simulink model "Regulation_Case"  (R2021a)
settings: Solver=VariableStepAuto  StartTime=0.0  StopTime=300  RelTol=1e-3
values from neighbouring files (symbols this model uses):
  kd = 500    [Parameters.m]
  kp = 50    [Parameters.m]
  omega0 = pi/180*[0.53 0.53 0.053]'    [Parameters.m]
  q0 = [0.6853 0.6953 0.1531 0.1531]'    [Parameters.m]
  qc = [0 0 0 1]'    [Parameters.m]
settings Model: Creator=VTX  LastModifiedBy=VTX

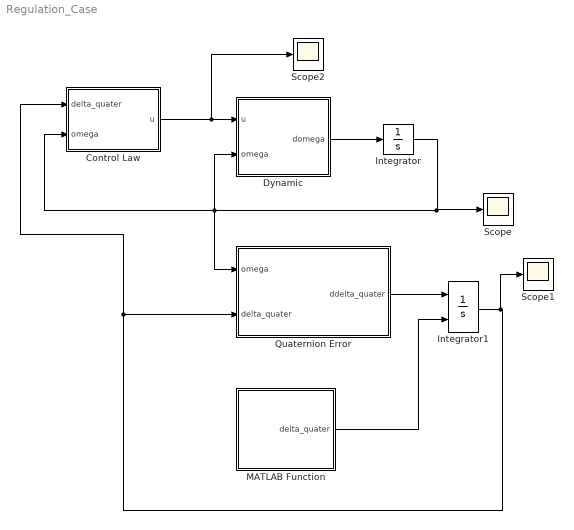
== system Regulation_Case ==
  Control Law : MATLAB Function  TreatAsAtomicUnit=on
  Dynamic : MATLAB Function  TreatAsAtomicUnit=on
  Integrator : Integrator  InitialCondition=omega0
  Integrator1 : Integrator  InitialConditionSource=external
  MATLAB Function : MATLAB Function  TreatAsAtomicUnit=on
  Quaternion Error : MATLAB Function  TreatAsAtomicUnit=on
  Scope : Scope
  Scope1 : Scope
  Scope2 : Scope
  wires:
  Control Law/1(u) -> Scope2/1, Dynamic/1(u)
  Dynamic/1(domega) -> Integrator/1
  Quaternion Error/1(ddelta_quater) -> Integrator1/1
  MATLAB Function/1(delta_quater) -> Integrator1/2
  Integrator1/1 -> Scope1/1, Control Law/1(delta_quater), Quaternion Error/2(delta_quater)
  Integrator/1 -> Scope/1, Control Law/2(omega), Quaternion Error/1(omega), Dynamic/2(omega)

== matlab function Regulation_Case/MATLAB Function ==
  data: delta_quater output; q0 parameter; qc parameter
function delta_quater = fcn(q0, qc)
    delta_quater_1to3 = property_matrix(qc)'*q0;
    delta_quater4 = q0'*qc;
    
    delta_quater = [delta_quater_1to3' delta_quater4]';
end

== matlab function Regulation_Case/Dynamic ==
  data: u input; domega output; omega input; J parameter
function domega = fcn(u,omega, J)
    domega = -inv(J)*(cross_matrix(omega)*J*omega - u);
end

== matlab function Regulation_Case/Control Law ==
  data: delta_quater input; u output; omega input; kp parameter; kd parameter
function u = fcn(delta_quater,omega, kp, kd)
    %u = -kp*delta_quater(1:3) - kd*(1 + delta_quater(1:3)'*delta_quater(1:3))*omega;
    u = -kp*delta_quater(1:3) - kd*omega;
end

== matlab function Regulation_Case/Quaternion Error ==
  data: ddelta_quater output; omega input; delta_quater input
function ddelta_quater = fcn(omega, delta_quater)
    ddelta_quater_1to3 = (cross_matrix(delta_quater(1:3))*omega + delta_quater(4)*omega)/2;
    ddelta_quater4 = -0.5*delta_quater(1:3)'*omega;
    
    ddelta_quater = [ddelta_quater_1to3' ddelta_quater4]';
end
